simulink model "Lab2"  (R2022a)
settings: Solver=ode23t  StartTime=0.0  StopTime=1  MaxStep=1e-5  RelTol=1e-3
values from neighbouring files (symbols this model uses):
  J = J1    (= 0.00035)    [LAB2.m]
  La = 0.00035    [LAB2.m]
  psi = 0.28648    [LAB2.m]
  Ra = 0.35    [LAB2.m]
  T_L = 0.68755    [LAB2.m]
  U = 12    [LAB2.m]
libraries: fl_lib x7, nesl_utility x5, ee_lib x1
settings Model: Creator=Troyeee  LastModifiedBy=81502
settings ModelReferenceCC: EnableRefExpFcnMdlSchedulingChecks=off
settings RTWCC: Description=Generic Real-Time Target  GPUComputeCapability=5.0

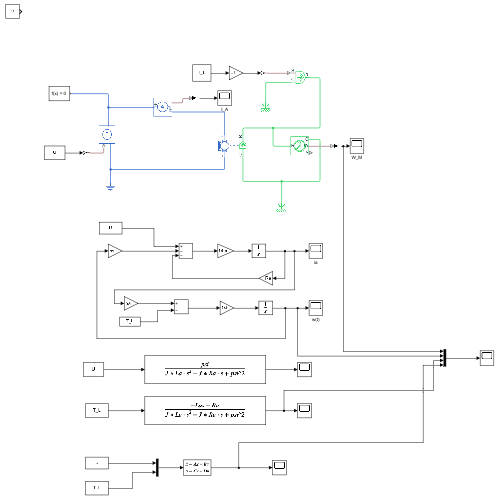
[thumbnail: Simulink's stored preview of the top-level diagram]
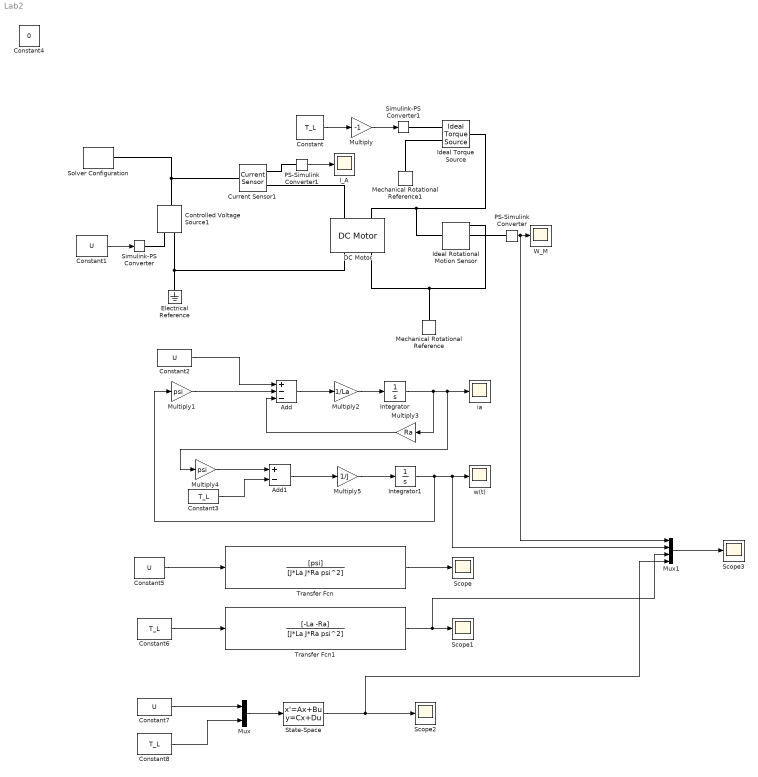
== system Lab2 ==
  Add : Sum  Inputs=+--
  Add1 : Sum  Inputs=+-
  Constant{,3,6,8} (4 alike) : Constant  Value=T_L
  Constant{1..2,5,7} (4 alike) : Constant  Value=U
  Constant4 : Constant  Value=0
  Controlled Voltage Source1 : fl_lib/Electrical/Electrical Sources/Controlled Voltage Source
      settings: SourceProductBaseCode=PW,SS,VE
  Current Sensor1 : fl_lib/Electrical/Electrical Sensors/Current Sensor
      settings: SourceProductBaseCode=PW,SS,VE
  DC Motor : ee_lib/Electromechanical/Brushed Motors/DC Motor  field_option=ee.enum.field_option.pm  Rf=100 Ohm  Lf=1 H  Laf=0.15 H  If0=0 A  parameterization=ee.enum.dcparam_option.circuit_param  Ra=Ra Ohm  La=La H  emf_or_torque=ee.enum.emf_or_torque.kv  Kv=psi V*s/rad  Ki=6.876e-4 N*m/A  T_stall=0.24e-3 N*m  w_max=19100 rpm  w_rated=15000 rpm  P_rated=0.08 W  V_rated=1.5 V  lam_param=ee.enum.lam_param.damping  i_noload=0 A  V_i_noload=1.5 V  J=J kg*m^2  lam=0 N*m*s/rad  speed0=0 rpm  enable_fault_armature=simscape.enum.onoff.off  rev_faulted=1 / 3  G_faulted_armature=1e-5 S  fault_trigger_armature=ee.enum.faults.faultTrigger.temporal  t_fault_armature=1 s  max_permissible_current_armature=inf A  t_fail_on_current_armature=1 s  enable_fault_field=simscape.enum.onoff.off  G_faulted_field=1e-5 S  fault_trigger_field=ee.enum.faults.faultTrigger.temporal  t_fault_field=1 s  max_permissible_current_field=inf A  t_fail_on_current_field=1 s  fault_action=simscape.enum.assert.action.none  alpha=3.93e-3 1/K  Tmeas=25 degC  thermal_mass=100 J/K  initial_temperature=25 degC
  Electrical Reference : fl_lib/Electrical/Electrical Elements/Electrical Reference
      settings: SourceProductBaseCode=PW,SS,VE
  I_A : Scope
  Ideal Rotational Motion Sensor : fl_lib/Mechanical/Mechanical Sensors/Ideal Rotational Motion Sensor  wrap_angle=false  offset=0 rad
      settings: SourceProductBaseCode=PW,SS,VE
  Ideal Torque Source : fl_lib/Mechanical/Mechanical Sources/Ideal Torque Source
      settings: SourceProductBaseCode=PW,SS,VE
  Integrator : Integrator
  Integrator1 : Integrator
  Mechanical Rotational Reference : fl_lib/Mechanical/Rotational Elements/Mechanical Rotational Reference
      settings: SourceProductBaseCode=PW,SS,VE
  Mechanical Rotational Reference1 : fl_lib/Mechanical/Rotational Elements/Mechanical Rotational Reference
      settings: SourceProductBaseCode=PW,SS,VE
  Multiply : Gain  Gain=-1
  Multiply1 : Gain  Gain=psi
  Multiply2 : Gain  Gain=1/La
  Multiply3 : Gain  Gain=Ra
  Multiply4 : Gain  Gain=psi
  Multiply5 : Gain  Gain=1/J
  Mux : Mux  Inputs=2
  Mux1 : Mux
  PS-Simulink Converter : nesl_utility/PS-Simulink Converter  PhysicalDomain=network_engine_domain  SubClassName=ps_output  LeftPortType=input  RightPortType=output  PseudoPeriodic=off  Frequencies=[]  VectorFormat=inherit  Unit=inherit  AffineConversion=off
      settings: SourceProductBaseCode=SS,PW,VE
  PS-Simulink Converter1 : nesl_utility/PS-Simulink Converter  PhysicalDomain=network_engine_domain  SubClassName=ps_output  LeftPortType=input  RightPortType=output  PseudoPeriodic=off  Frequencies=[]  VectorFormat=inherit  Unit=inherit  AffineConversion=off
      settings: SourceProductBaseCode=SS,PW,VE
  Scope{,1..3} (4 alike) : Scope
  Simulink-PS Converter : nesl_utility/Simulink-PS Converter  PhysicalDomain=network_engine_domain  SubClassName=ps_input  LeftPortType=input  RightPortType=output  PseudoPeriodic=off  Frequencies=[]  NoiseDistribution=none  NoiseParameters=[]  Unit=1  AffineConversion=off  FilteringAndDerivatives=provide  SimscapeFilterOrder=1  InputFilterTimeConstant=0.001  UdotUserProvided=0
      settings: SourceProductBaseCode=SS,PW,VE
  Simulink-PS Converter1 : nesl_utility/Simulink-PS Converter  PhysicalDomain=network_engine_domain  SubClassName=ps_input  LeftPortType=input  RightPortType=output  PseudoPeriodic=off  Frequencies=[]  NoiseDistribution=none  NoiseParameters=[]  Unit=1  AffineConversion=off  FilteringAndDerivatives=provide  SimscapeFilterOrder=1  InputFilterTimeConstant=0.001  UdotUserProvided=0
      settings: SourceProductBaseCode=SS,PW,VE
  Solver Configuration : nesl_utility/Solver Configuration  PhysicalDomain=network_engine_domain  SubClassName=solver  LeftPortType=input  RightPortType=generic  Tones=[]  Harmonics=[]  SimulateNoise=off  Profile=off  UseLocalSampling=off  EnableSwitchedLinearOptims=on  FrequencyDomain=off  UseCCode=off  RelTol=0.001  AbsTol=0.001  MinStep=1e-09  ToWorkspace=off  RevertToSquareIcSolve=off  NumHomotopyIterations=100  PhasorMode=off  PhasorModeNumHarmonics=1  IndexReductionMethod=DerivativeReplacement  DoDC=off  ResidualTolerance=1e-09  UseLocalSolver=off  LocalSolverChoice=NE_BACKWARD_EULER_ADVANCER  LocalSolverSampleTime=0.001  DoFixedCost=off  MaxNonlinIter=3  MaxModeIter=2  ComputeImpulses=off  ImpulseIterations=2  LinearAlgebra=auto  LinearAlgebraNumThread=0  EquationFormulation=NE_TIME_EF  DelaysMemoryBudget=1024  AutomaticFiltering=on  FilteringTimeConstant=0.001  PartitionStorageMethod=AS_NEEDED  PartitionMemoryBudget=1024  PartitionMethod=ROBUST
      settings: SourceProductBaseCode=SS,PW,VE
  State-Space : StateSpace  A=[-Ra/La -psi/La;psi/J 0]  B=[1/La 0;0 -1/J]  C=[0 1]  D=[0 0]  InitialCondition=0
  Transfer Fcn : TransferFcn  Numerator=[psi]  Denominator=[J*La J*Ra psi^2]
  Transfer Fcn1 : TransferFcn  Numerator=[-La -Ra]  Denominator=[J*La J*Ra psi^2]
  W_M : Scope
  ia : Scope
  w(t) : Scope
  wires:
  Constant1/1 -> Simulink-PS Converter/1
  Multiply/1 -> Simulink-PS Converter1/1
  PS-Simulink Converter1/1 -> I_A/1
  Constant2/1 -> Add/1
  Multiply1/1 -> Add/2
  Add/1 -> Multiply2/1
  Multiply2/1 -> Integrator/1
  Integrator/1 -> Multiply3/1, Multiply4/1, ia/1
  Multiply3/1 -> Add/3
  Multiply4/1 -> Add1/1
  Constant3/1 -> Add1/2
  Add1/1 -> Multiply5/1
  Multiply5/1 -> Integrator1/1
  Integrator1/1 -> Multiply1/1, Mux1/2, w(t)/1
  Constant/1 -> Multiply/1
  Constant5/1 -> Transfer Fcn/1
  Constant6/1 -> Transfer Fcn1/1
  Transfer Fcn1/1 -> Mux1/3, Scope1/1
  Constant7/1 -> Mux/1
  Constant8/1 -> Mux/2
  Mux/1 -> State-Space/1
  State-Space/1 -> Mux1/4, Scope2/1
  PS-Simulink Converter/1 -> Mux1/1, W_M/1
  Mux1/1 -> Scope3/1
  Transfer Fcn/1 -> Scope/1
  connections:
  Solver Configuration/RConn1 -- Current Sensor1/LConn1 -- Controlled Voltage Source1/LConn1
  Simulink-PS Converter/RConn1 -- Controlled Voltage Source1/RConn1
  Electrical Reference/LConn1 -- DC Motor/RConn1 -- Controlled Voltage Source1/RConn2
  Current Sensor1/RConn2 -- DC Motor/LConn1
  Mechanical Rotational Reference/LConn1 -- DC Motor/RConn2 -- Ideal Rotational Motion Sensor/RConn1
  PS-Simulink Converter/LConn1 -- Ideal Rotational Motion Sensor/RConn2
  Ideal Torque Source/RConn2 -- Mechanical Rotational Reference1/LConn1
  Ideal Torque Source/LConn1 -- Ideal Rotational Motion Sensor/LConn1 -- DC Motor/LConn2
  Simulink-PS Converter1/RConn1 -- Ideal Torque Source/RConn1
  PS-Simulink Converter1/LConn1 -- Current Sensor1/RConn1
